simulink model "BlokSchema"  (R2023b)
settings: Solver=VariableStepAuto  StartTime=0.0  StopTime=5000  RelTol=1e-5
values from neighbouring files (symbols this model uses):
  citatel = (K/(T1*T2))    (= 0.00186096256684)    [Zadanie4.m]
  Delay = 300    [Zadanie4.m]
  menovatel = [1,(T1+T2)/(T1*T2), 1/(T1*T2)]    [Zadanie4.m]
  q00 = P*(1+(Td/T)+(T/Ti))    [Zadanie4.m]
  q11 = (-P*(1+((2*Td)/T)))    [Zadanie4.m]
  q22 = ((P*Td)/T)    [Zadanie4.m]
  T = 300    [Zadanie4.m]
undefined symbols (not defined in the file or in its folder): p11, p12, p13, q10, q12, q13
settings Model: PacingRate=1000  Creator=domin  LastModifiedBy=domin

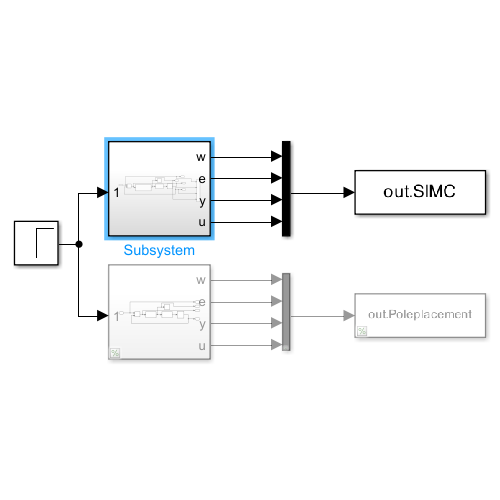
[thumbnail: Simulink's stored preview of the top-level diagram]
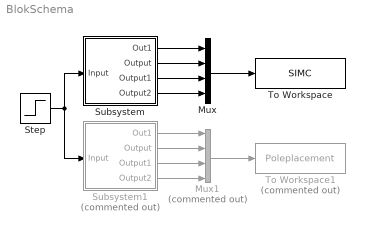
== system BlokSchema ==
  Mux : Mux
  Mux1 : Mux  Commented=on
  Step : Step  Time=0  Before=1  SampleTime=0
  Subsystem : Subsystem
  Subsystem1 : Subsystem  Commented=on
  To Workspace : ToWorkspace  VariableName=SIMC  SaveFormat=Timeseries  SampleTime=-1
  To Workspace1 : ToWorkspace  Commented=on  VariableName=Poleplacement  SampleTime=-1
  wires:
  Step/1 -> Subsystem/1(Input), Subsystem1/1(Input)
  Subsystem/1(Out1) -> Mux/1
  Subsystem/2(Output) -> Mux/2
  Subsystem/3(Output1) -> Mux/3
  Subsystem/4(Output2) -> Mux/4
  Mux/1 -> To Workspace/1
  Mux1/1 -> To Workspace1/1
  Subsystem1/1(Out1) -> Mux1/1
  Subsystem1/2(Output) -> Mux1/2
  Subsystem1/3(Output1) -> Mux1/3
  Subsystem1/4(Output2) -> Mux1/4

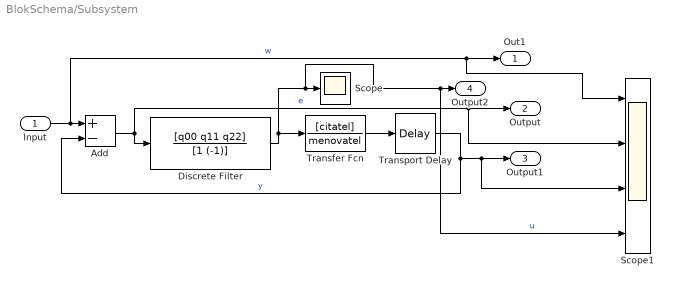
== system BlokSchema/Subsystem ==
  Input : Inport
  Add : Sum  Inputs=+-
  Discrete Filter : DiscreteFilter  Numerator=[q00 q11 q22]  Denominator=[1 (-1)]  SampleTime=T
  Scope : Scope
  Scope1 : Scope  NumInputPorts=4
  Transfer Fcn : TransferFcn  Numerator=[citatel]  Denominator=menovatel
  Transport Delay : TransportDelay  DelayTime=Delay
  Out1 : Outport
  Output : Outport  Port=2
  Output1 : Outport  Port=3
  Output2 : Outport  Port=4
  wires:
  Add/1 -> Scope1/2, Output/1, Discrete Filter/1  "e"
  Input/1 -> Scope1/1, Out1/1, Add/1  "w"
  Transfer Fcn/1 -> Transport Delay/1
  Discrete Filter/1 -> Transfer Fcn/1, Scope1/4, Output2/1, Scope/1  "u"
  Transport Delay/1 -> Scope1/3, Output1/1, Add/2  "y"

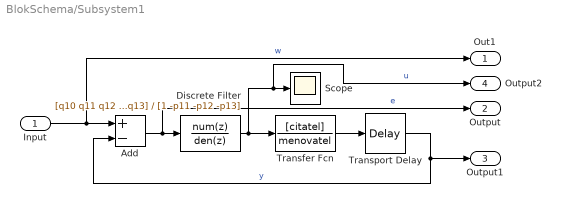
== system BlokSchema/Subsystem1 ==
  Input : Inport
  Add : Sum  Inputs=+-
  Discrete Filter : DiscreteFilter  Numerator=[q10 q11 q12 q13]  Denominator=[1 -p11 -p12 -p13]  SampleTime=T
  Scope : Scope
  Transfer Fcn : TransferFcn  Numerator=[citatel]  Denominator=menovatel
  Transport Delay : TransportDelay  DelayTime=Delay
  Out1 : Outport
  Output : Outport  Port=2
  Output1 : Outport  Port=3
  Output2 : Outport  Port=4
  wires:
  Add/1 -> Discrete Filter/1, Output/1  "e"
  Input/1 -> Out1/1, Add/1  "w"
  Transfer Fcn/1 -> Transport Delay/1
  Discrete Filter/1 -> Transfer Fcn/1, Output2/1, Scope/1  "u"
  Transport Delay/1 -> Output1/1, Add/2  "y"
